simulink model "motor_control_with_off_the_shelf_SVPWM"  (Simulink 7.9)
settings: Solver=ode45  StartTime=0.0  StopTime=1  RelTol=1e-3
libraries: powerlib x10, simulink x3, powerlib_extras x1
settings Model: Creator=Dmitriy  LastModifiedBy=Dmitriy
settings GRTTargetCC: CombineOutputUpdateFcns=off  GRTInterface=on

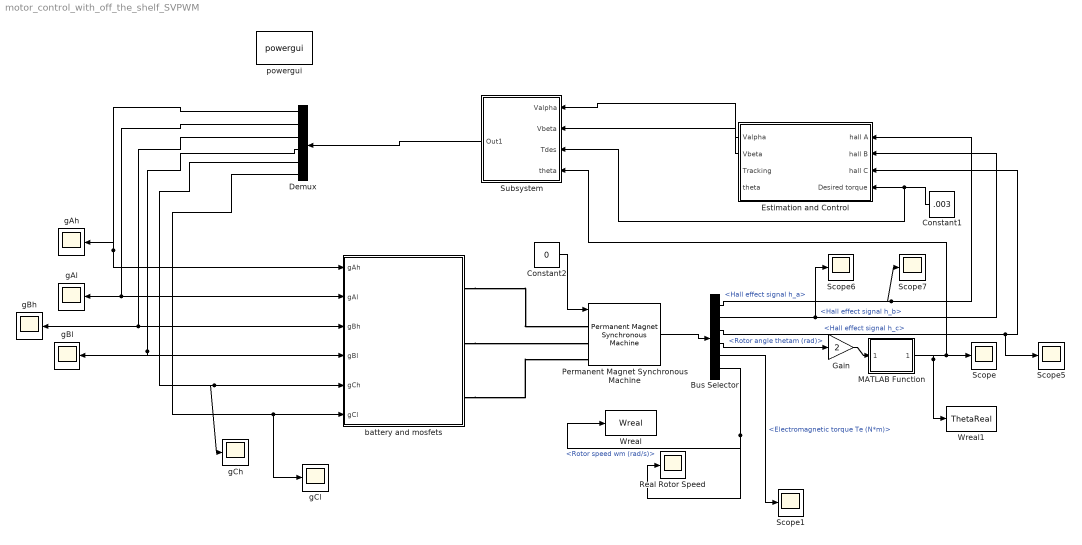
== system motor_control_with_off_the_shelf_SVPWM ==
  Bus Selector : BusSelector  OutputSignals=Hall effect signal h_a,Hall effect signal h_b,Hall effect signal h_c,Rotor angle thetam (rad),Electromagnetic torque Te (N*m),Rotor speed wm (rad/s)
  Constant1 : Constant  Value=.003
  Constant2 : Constant  Value=0
  Demux : Demux  Outputs=6
  Estimation and Control : Subsystem  SystemSampleTime=.001
  Gain : Gain  Gain=2
  MATLAB Function : MATLAB Function  TreatAsAtomicUnit=on
  Permanent Magnet Synchronous Machine : powerlib/Machines/Permanent Magnet Synchronous Machine  NbPhases=3  FluxDistribution=Sinusoidal  RotorType=Round  MechanicalLoad=Torque Tm  PresetModel=No  ShowDetailedParameters=on  Resistance=28.2  Inductance=8.5e-3  dqInductances=[0.006365 0.006365]  La=1940*10^-6  MachineConstant=Torque Constant (N.m / A_peak)  Flux=0.0060333  VoltageCst=2.1887  TorqueCst=0.0181  Flat=120  Mechanical=[0.0001 5.396e-005 2 0]  PolePairs=2  InitialConditions=[0,1, 0,0]  InitialConditions5ph=[0 0 0 0 0 0]  TsPowergui=0  TsBlock=-1  RefAngle=Aligned with phase A axis (original Park)
  Real Rotor Speed : Scope
      settings: YMin=9.27  YMax=9.44  SaveName=ScopeData18
  Scope{,1,5..7} (5 alike) : Scope
      Scope settings: YMin=4.005  YMax=4.115
      Scope1 settings: YMin=-1e-05  YMax=0.00013
      Scope5 settings: SaveName=ScopeData5
      Scope6 settings: SaveName=ScopeData6
      Scope7 settings: SaveName=ScopeData7
  Subsystem : Subsystem
  Wreal : ToWorkspace  VariableName=Wreal  SampleTime=-1  SaveFormat=Timeseries
  Wreal1 : ToWorkspace  VariableName=ThetaReal  SampleTime=-1  SaveFormat=Timeseries
  battery and mosfets : Subsystem
  gAh : Scope
      settings: SaveName=ScopeData11
  gAl : Scope
      settings: SaveName=ScopeData10
  gBh : Scope
      settings: SaveName=ScopeData9
  gBl : Scope
      settings: SaveName=ScopeData8
  gCh : Scope
      settings: YMin=0.95  YMax=1.05  SaveName=ScopeData4
  gCl : Scope
      settings: YMin=0.95  YMax=1.05  SaveName=ScopeData2
  powergui : powerlib/powergui  Priority=1  SimulationMode=Continuous  SolverType=Tustin  SampleTime=50e-6  frequency=60  SPID=off  DisableSnubberDevices=off  DisableRonSwitches=off  DisableVfSwitches=off  SwTol=0  Interpol=off  DisplayEquations=off  FunctionMessages=off  frequencyindice=0  Pbase=100e6  ErrMax=1e-4  Iterations=50  UnitsV=kV  UnitsW=MW  echomessages=off  HookPort=off  EnableUseOfTLC=off  x0status=blocks  RestoreLinks=warning  ResistiveCurrentMeasurement=off  Ylog=off  Xlog=on  ShowGrid=off  save=off  variable=ZData  ZoomFFT=off  StartTime=0.0  cycles=1  DisplayStyle=1  FreqAxis=off  MaxFrequency=1000  frequencyindicesteady=1  display=off  methode=off
  wires:
  Permanent Magnet Synchronous Machine/1 -> Bus Selector/1
  Bus Selector/1 -> Estimation and Control/1(hall A), Scope7/1  "<Hall effect signal h_a>"
  Bus Selector/3 -> Estimation and Control/3(hall C), Scope5/1  "<Hall effect signal h_c>"
  Bus Selector/4 -> Gain/1  "<Rotor angle thetam (rad)>"
  Bus Selector/5 -> Scope1/1  "<Electromagnetic torque Te (N*m)>"
  Bus Selector/2 -> Estimation and Control/2(hall B), Scope6/1  "<Hall effect signal h_b>"
  Demux/6 -> battery and mosfets/6(gCl), gCl/1
  Demux/5 -> battery and mosfets/5(gCh), gCh/1
  Demux/4 -> battery and mosfets/4(gBl), gBl/1
  Demux/3 -> battery and mosfets/3(gBh), gBh/1
  Demux/2 -> battery and mosfets/2(gAl), gAl/1
  Demux/1 -> battery and mosfets/1(gAh), gAh/1
  Constant1/1 -> Estimation and Control/4(Desired torque), Subsystem/3(Tdes)
  Bus Selector/6 -> Real Rotor Speed/1, Wreal/1  "<Rotor speed wm (rad/s)>"
  MATLAB Function/1(lambda1) -> Wreal1/1, Scope/1, Subsystem/4(theta)
  Gain/1 -> MATLAB Function/1(lambda)
  Constant2/1 -> Permanent Magnet Synchronous Machine/1
  Estimation and Control/1(Valpha) -> Subsystem/1(Valpha)
  Estimation and Control/2(Vbeta) -> Subsystem/2(Vbeta)
  Subsystem/1(Out1) -> Demux/1
  connections:
  battery and mosfets/RConn1 -- Permanent Magnet Synchronous Machine/LConn1
  battery and mosfets/RConn2 -- Permanent Magnet Synchronous Machine/LConn2
  battery and mosfets/RConn3 -- Permanent Magnet Synchronous Machine/LConn3

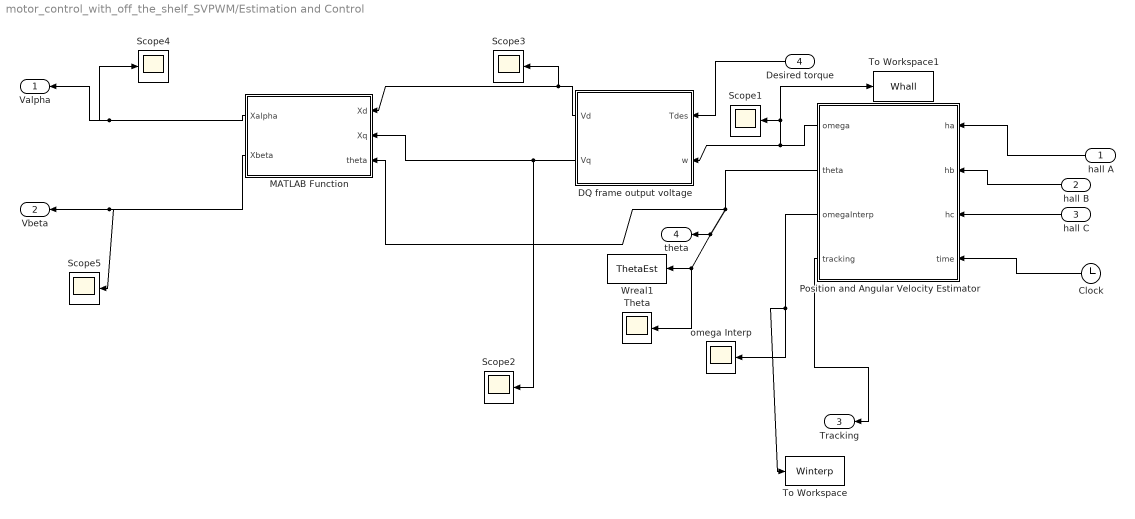
== system motor_control_with_off_the_shelf_SVPWM/Estimation and Control ==
  hall A : Inport
  hall B : Inport  Port=2
  hall C : Inport  Port=3
  Desired torque : Inport  Port=4
  Clock : Clock
  DQ frame output voltage : MATLAB Function  TreatAsAtomicUnit=on  SystemSampleTime=.0001
  MATLAB Function : MATLAB Function  TreatAsAtomicUnit=on
  Position and Angular Velocity Estimator : MATLAB Function  TreatAsAtomicUnit=on  SystemSampleTime=.0001
  Scope{1..5} (5 alike) : Scope
      Scope1 settings: SaveName=ScopeData13
      Scope2 settings: SaveName=ScopeData14
      Scope3 settings: SaveName=ScopeData15
      Scope4 settings: SaveName=ScopeData16
      Scope5 settings: SaveName=ScopeData17
  Theta : Scope
      settings: YMin=5.75959  YMax=5.75959  SaveName=ScopeData12
  To Workspace : ToWorkspace  VariableName=Winterp  SampleTime=-1  SaveFormat=Timeseries
  To Workspace1 : ToWorkspace  VariableName=Whall  SampleTime=-1  SaveFormat=Timeseries
  Wreal1 : ToWorkspace  VariableName=ThetaEst  SampleTime=-1  SaveFormat=Timeseries
  omega Interp : Scope
      settings: YMin=0  YMax=3.25  SaveName=ScopeData19
  Valpha : Outport
  Vbeta : Outport  Port=2
  Tracking : Outport  Port=3
  theta : Outport  Port=4
  wires:
  Position and Angular Velocity Estimator/1(omega) -> DQ frame output voltage/2(w), Scope1/1, To Workspace1/1
  Desired torque/1 -> DQ frame output voltage/1(Tdes)
  hall A/1 -> Position and Angular Velocity Estimator/1(ha)
  hall B/1 -> Position and Angular Velocity Estimator/2(hb)
  hall C/1 -> Position and Angular Velocity Estimator/3(hc)
  Position and Angular Velocity Estimator/2(theta) -> MATLAB Function/3(theta), Theta/1, Wreal1/1, theta/1
  DQ frame output voltage/2(Vq) -> Scope2/1, MATLAB Function/2(Xq)
  DQ frame output voltage/1(Vd) -> Scope3/1, MATLAB Function/1(Xd)
  MATLAB Function/1(Xalpha) -> Valpha/1, Scope4/1
  MATLAB Function/2(Xbeta) -> Vbeta/1, Scope5/1
  Position and Angular Velocity Estimator/3(omegaInterp) -> omega Interp/1, To Workspace/1
  Clock/1 -> Position and Angular Velocity Estimator/4(time)
  Position and Angular Velocity Estimator/4(tracking) -> Tracking/1

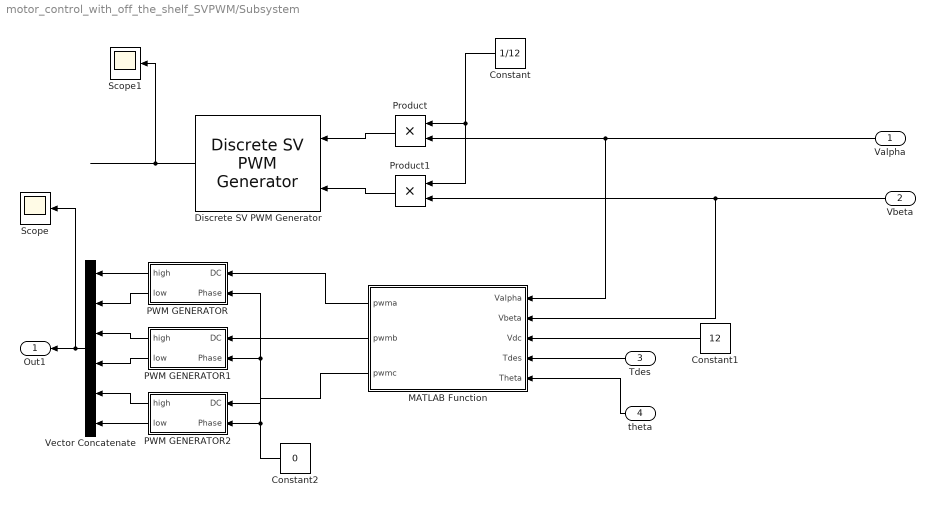
== system motor_control_with_off_the_shelf_SVPWM/Subsystem ==
  Valpha : Inport
  Vbeta : Inport  Port=2
  Tdes : Inport  Port=3
  theta : Inport  Port=4
  Constant : Constant  Value=1/12
  Constant1 : Constant  Value=12
  Constant2 : Constant  Value=0
  Discrete SV PWM Generator : powerlib_extras/Discrete  Control Blocks/Discrete SV PWM Generator  InputType=alpha-beta components  SwitchingPattern=Pattern #1  Fc=2000  ParUref=[0.8 -30 50]  Ts=2e-6
  MATLAB Function : MATLAB Function  TreatAsAtomicUnit=on
  PWM GENERATOR : Subsystem  TreatAsAtomicUnit=on  SystemSampleTime=10^-6
      settings: ErrorFcn=10^6
  PWM GENERATOR1 : Subsystem  TreatAsAtomicUnit=on  SystemSampleTime=10^-6
  PWM GENERATOR2 : Subsystem  TreatAsAtomicUnit=on  SystemSampleTime=10^-6
  Product : Product  RndMeth=Zero
  Product1 : Product  RndMeth=Zero
  Scope : Scope
      settings: SaveName=ScopeData3
  Scope1 : Scope
      settings: SaveName=ScopeData20
  Vector Concatenate : Concatenate  NumInputs=6
  Out1 : Outport
  wires:
  Constant/1 -> Product/1, Product1/1
  Product/1 -> Discrete SV PWM Generator/1
  Product1/1 -> Discrete SV PWM Generator/2
  Valpha/1 -> Product/2, MATLAB Function/1(Valpha)
  Discrete SV PWM Generator/1 -> Scope1/1
  Vbeta/1 -> Product1/2, MATLAB Function/2(Vbeta)
  Constant1/1 -> MATLAB Function/3(Vdc)
  Tdes/1 -> MATLAB Function/4(Tdes)
  theta/1 -> MATLAB Function/5(Theta)
  MATLAB Function/2(pwmb) -> PWM GENERATOR1/1(DC)
  MATLAB Function/3(pwmc) -> PWM GENERATOR2/1(DC)
  MATLAB Function/1(pwma) -> PWM GENERATOR/1(DC)
  Constant2/1 -> PWM GENERATOR2/2(Phase), PWM GENERATOR1/2(Phase), PWM GENERATOR/2(Phase)
  PWM GENERATOR/1(high) -> Vector Concatenate/1
  PWM GENERATOR/2(low) -> Vector Concatenate/2
  PWM GENERATOR1/1(high) -> Vector Concatenate/3
  PWM GENERATOR1/2(low) -> Vector Concatenate/4
  PWM GENERATOR2/1(high) -> Vector Concatenate/5
  PWM GENERATOR2/2(low) -> Vector Concatenate/6
  Vector Concatenate/1 -> Out1/1, Scope/1

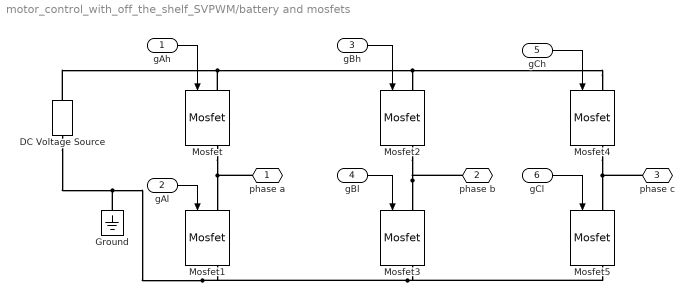
== system motor_control_with_off_the_shelf_SVPWM/battery and mosfets ==
  gAh : Inport
  gAl : Inport  Port=2
  gBh : Inport  Port=3
  gBl : Inport  Port=4
  gCh : Inport  Port=5
  gCl : Inport  Port=6
  DC Voltage Source : powerlib/Electrical Sources/DC Voltage Source  Amplitude=12  Measurements=None
  Ground : powerlib/Elements/Ground  LConnTagsString=a
  Mosfet{,1..5} (6 alike) : powerlib/Power Electronics/Mosfet  Ron=0.1  Lon=0  Rd=0.01  Vfd=0  IC=0  Rs=1e5  Cs=inf  Measurements=on
  phase a : PMIOPort  Port=1  Side=Right
  phase b : PMIOPort  Port=2  Side=Right
  phase c : PMIOPort  Port=3  Side=Right
  wires:
  gCl/1 -> Mosfet5/1
  gCh/1 -> Mosfet4/1
  gBh/1 -> Mosfet2/1
  gBl/1 -> Mosfet3/1
  gAl/1 -> Mosfet1/1
  gAh/1 -> Mosfet/1
  connections:
  Mosfet/RConn1 -- Mosfet1/LConn1 -- phase a/RConn1
  Mosfet2/RConn1 -- Mosfet3/LConn1 -- phase b/RConn1
  phase c/RConn1 -- Mosfet4/RConn1 -- Mosfet5/LConn1
  Mosfet1/RConn1 -- Ground/LConn1 -- DC Voltage Source/LConn1 -- Mosfet3/RConn1 -- Mosfet5/RConn1
  Mosfet4/LConn1 -- Mosfet/LConn1 -- DC Voltage Source/RConn1 -- Mosfet2/LConn1

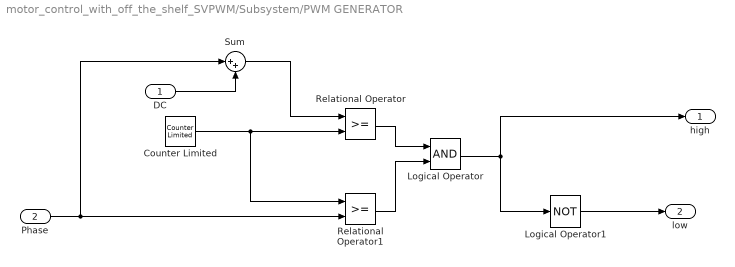
== system motor_control_with_off_the_shelf_SVPWM/Subsystem/PWM GENERATOR ==
  DC : Inport
  Phase : Inport  Port=2
  Counter Limited : simulink/Sources/Counter Limited  uplimit=1000  tsamp=-1
  Logical Operator : Logic  AllPortsSameDT=off  OutDataTypeStr=boolean
  Logical Operator1 : Logic  Operator=NOT  AllPortsSameDT=off  OutDataTypeStr=boolean
  Relational Operator : RelationalOperator  OutDataTypeStr=boolean
  Relational Operator1 : RelationalOperator  OutDataTypeStr=boolean
  Sum : Sum  Inputs=|++
  high : Outport
  low : Outport  Port=2
  wires:
  Counter Limited/1 -> Relational Operator/2, Relational Operator1/1
  Phase/1 -> Relational Operator1/2, Sum/1
  DC/1 -> Sum/2
  Sum/1 -> Relational Operator/1
  Relational Operator/1 -> Logical Operator/1
  Relational Operator1/1 -> Logical Operator/2
  Logical Operator/1 -> Logical Operator1/1, high/1
  Logical Operator1/1 -> low/1

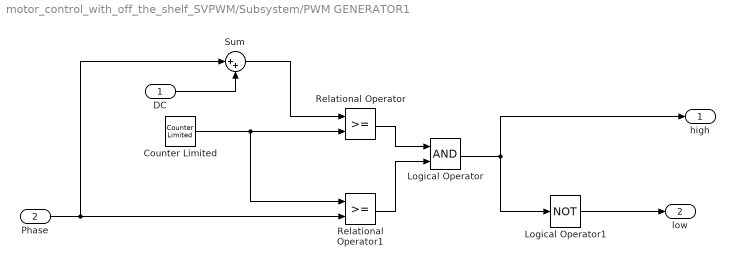
== system motor_control_with_off_the_shelf_SVPWM/Subsystem/PWM GENERATOR1 ==
  DC : Inport
  Phase : Inport  Port=2
  Counter Limited : simulink/Sources/Counter Limited  uplimit=1000  tsamp=-1
  Logical Operator : Logic  AllPortsSameDT=off  OutDataTypeStr=boolean
  Logical Operator1 : Logic  Operator=NOT  AllPortsSameDT=off  OutDataTypeStr=boolean
  Relational Operator : RelationalOperator  OutDataTypeStr=boolean
  Relational Operator1 : RelationalOperator  OutDataTypeStr=boolean
  Sum : Sum  Inputs=|++
  high : Outport
  low : Outport  Port=2
  wires:
  Counter Limited/1 -> Relational Operator/2, Relational Operator1/1
  Phase/1 -> Relational Operator1/2, Sum/1
  DC/1 -> Sum/2
  Sum/1 -> Relational Operator/1
  Relational Operator/1 -> Logical Operator/1
  Relational Operator1/1 -> Logical Operator/2
  Logical Operator/1 -> Logical Operator1/1, high/1
  Logical Operator1/1 -> low/1

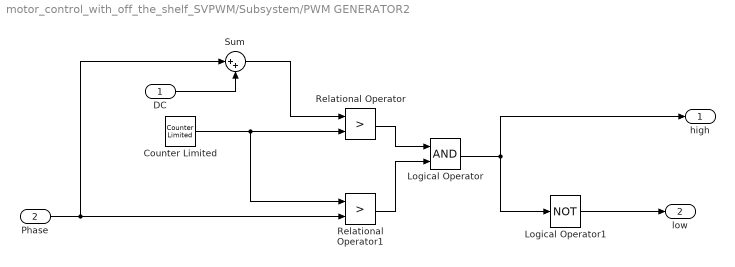
== system motor_control_with_off_the_shelf_SVPWM/Subsystem/PWM GENERATOR2 ==
  DC : Inport
  Phase : Inport  Port=2
  Counter Limited : simulink/Sources/Counter Limited  uplimit=1000  tsamp=-1
  Logical Operator : Logic  AllPortsSameDT=off  OutDataTypeStr=boolean
  Logical Operator1 : Logic  Operator=NOT  AllPortsSameDT=off  OutDataTypeStr=boolean
  Relational Operator : RelationalOperator  Operator=>  OutDataTypeStr=boolean
  Relational Operator1 : RelationalOperator  Operator=>  OutDataTypeStr=boolean
  Sum : Sum  Inputs=|++
  high : Outport
  low : Outport  Port=2
  wires:
  Counter Limited/1 -> Relational Operator/2, Relational Operator1/1
  Phase/1 -> Relational Operator1/2, Sum/1
  DC/1 -> Sum/2
  Sum/1 -> Relational Operator/1
  Relational Operator/1 -> Logical Operator/1
  Relational Operator1/1 -> Logical Operator/2
  Logical Operator/1 -> Logical Operator1/1, high/1
  Logical Operator1/1 -> low/1

== matlab function Estimation and Control/DQ frame output voltage ==
  data: Tdes input double; Vd output double; w input double; Vq output double
function [Vd,Vq] = computeDQOutput(Tdes,w)
%#codegen
%take the desired torque current 
% speed and compute the output voltage vector in the DQ
%frame. 

L = 1940*10^-6;
R = 28.2;
Ke = (1.895*10^-3)*9.54929659643; % convert to V/(rad/s) 
Kt = 1.81*10^3; %Nm/Amp

%because I is assumed to be on Q axis, T = KtI
Ides = Tdes/Kt;

%bemf is on q axis
bemf = Ke*w;

%inductor impedance 
ZL = L*w;

Vq = bemf+Ides*R;
Vd = -ZL*Ides;

== matlab function Estimation and Control/Position and Angular Velocity Estimator ==
  data: omega output double; ha input double; theta output double; hb input double; hc input double; omegaInterp output double; time input double; tracking output double
function [omega,theta, omegaInterp, tracking] = rotor_est(ha,hb,hc,time)
%#codegen

%estimate the position of the rotor in degrees electrical
%tracking is 0 or 1, 0 means the estimate is bad. Used for activating block
%commutation at initialization
omega=0;
theta=0;
omegaInterp = 0;
time
tracking =0;
coder.extrinsic('rotor_estimate');

[omega theta omegaInterp tracking] = rotor_estimate(ha,hb,hc,time);
end

== matlab function Subsystem/MATLAB Function ==
  data: Valpha input double; pwma output double; Vbeta input double; Vdc input double; Tdes input double; Theta input double; pwmb output double; pwmc output double
function [pwma,pwmb,pwmc]  = block_com(Valpha,Vbeta,Vdc,Tdes,Theta)
%#codegen

ang = floor(Theta/(pi/3));

d = sqrt(Valpha^2+Vbeta^2)/Vdc;
d = 1;


switch ang
    case 0
        if(Tdes>=0)
            %s2
            pwms = [d d 0];
        else
            %s1
            pwms = [d 0 0];
        end
    case 1
        if(Tdes>=0)
            %s3
            pwms = [0 d 0];
        else
            %s2
            pwms = [d d 0];
        end
        
    case 2
        if(Tdes>=0)
            %s4
            pwms = [0 d d];
        else
            %s3
            pwms = [0 d 0];
        end
    case 3
        if(Tdes>=0)
            %s5
            pwms = [0 0 d];
        else
            %s4
            pwms = [0 d d];
        end
    case 4
        if(Tdes>=0)
            %s6
            pwms = [d 0 d];
        else
            %s5
            pwms = [0 0 d];
        end
    case 5
        if(Tdes>=0)
            %s1
            pwms = [d 0 0];
        else
            %s6
            pwms = [d 0 d];
        end
        
    otherwise
        pwms = [0 0 0];
end
pwms=pwms*1000;
pwma=pwms(1);
pwmb= pwms(2);
pwmc = pwms(3);

== matlab function MATLAB Function ==
  data: lambda input double; lambda1 output double
function lambda1 = wrapTo2Pi(lambda)
%wrapTo2Pi Wrap angle in radians to [0 2*pi]
%
%   lambdaWrapped = wrapTo2Pi(LAMBDA) wraps angles in LAMBDA, in radians,
%   to the interval [0 2*pi] such that zero maps to zero and 2*pi maps
%   to 2*pi. (In general, positive multiples of 2*pi map to 2*pi and
%   negative multiples of 2*pi map to zero.)
%
%   See also wrapToPi, wrapTo180, wrapTo360.

% Copyright 2007-2008 The MathWorks, Inc.
% $Revision: 1.1.6.1 $  $Date: 2008/12/22 23:50:53 $


positiveInput = (lambda > 0);
lambda = mod(lambda, 2*pi);
lambda((lambda == 0) & positiveInput) = 2*pi;
lambda1=lambda;
end

== matlab function Estimation and Control/MATLAB Function ==
  data: Xd input double; Xalpha output double; Xq input double; theta input double; Xbeta output double
function [Xalpha,Xbeta] = inversePark(Xd,Xq,theta)
%#codegen
%implements inverse park as described in james mevey's thesis

c = cos(theta);
s = sin(theta);

ipm = [c -s; s c];

xab = ipm*[Xd Xq]';

Xalpha = xab(1);
Xbeta = xab(2);
end
